simulink model "EXPDmodel"  (Simulink 8.3)
settings: Solver=ode3  StartTime=0.0  StopTime=3.999875  FixedStep=1/8000  RelTol=1e-3
values from neighbouring files (symbols this model uses):
  fa = 8000    [ExpA.m]
libraries: dspsrcs4 x1
settings Model: Creator=dsv1_5  LastModifiedBy=dsv1_5
settings DataIOCC: SignalLoggingSaveFormat=Dataset
settings DebuggingCC: UnderspecifiedInitializationDetection=Simplified  StateNameClashWarn=none
settings GRTTargetCC: CombineOutputUpdateFcns=on  GRTInterface=off

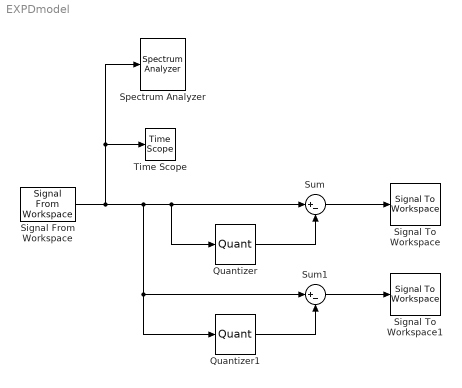
== system EXPDmodel ==
  Quantizer : Quantizer  QuantizationInterval=1/128  LinearizeAsGain=off
  Quantizer1 : Quantizer  QuantizationInterval=1/4  LinearizeAsGain=off
  Signal From Workspace : dspsrcs4/Signal From Workspace  X=signal2  Ts=1/fa  nsamps=1  OutputAfterFinalValue=Setting to zero  ignoreOrWarnInputAndFrameLengths=off
  Signal To Workspace : SignalToWorkspace  VariableName=noise128
      settings: CopyFcn=dspblkcopystw(gcbh);
  Signal To Workspace1 : SignalToWorkspace  VariableName=noise4
      settings: CopyFcn=dspblkcopystw(gcbh);
  Spectrum Analyzer : SpectrumAnalyzer  ScopeSpecification=DataTag0
  Sum : Sum  Inputs=|+-
  Sum1 : Sum  Inputs=|+-
  Time Scope : TimeScope  DefaultConfigurationName=spbscopes.TimeScopeBlockCfg  ScopeSpecification=DataTag1
  wires:
  Signal From Workspace/1 -> Time Scope/1, Spectrum Analyzer/1, Quantizer1/1, Sum1/1, Quantizer/1, Sum/1
  Sum/1 -> Signal To Workspace/1
  Quantizer/1 -> Sum/2
  Sum1/1 -> Signal To Workspace1/1
  Quantizer1/1 -> Sum1/2
